simulink model "sl_groundvehicleDynamics"  (R2022b)
settings: Solver=ode45  StartTime=0.0  StopTime=50  RelTol=1e-5  EnableMultiTasking=on
libraries: simulink x4, mobileRoboticsLib x3, simulink_extras x2
settings Model: Creator=sriramn  LastModifiedBy=n10474056
settings SolverCC: ZeroCrossAlgorithm=Adaptive  AlgebraicLoopSolver=TrustRegion
settings DataIOCC: LimitDataPoints=on  SaveFormat=Array  ReturnWorkspaceOutputs=off
settings OptimizationCC: LifeSpan=inf
settings DebuggingCC: SolverPrmCheckMsg=warning  UnconnectedInputMsg=warning  UnconnectedOutputMsg=warning  UnconnectedLineMsg=warning  AllowSymbolicDim=off  SFUnexpectedBacktrackingDiag=warning  SFNoUnconditionalDefaultTransitionDiag=warning  SFExecutionAtInitializationDiag=none  SFMachineParentedDataDiag=warning  ArithmeticOperatorsInVariantConditions=warning
settings HardwareCC: ProdBitPerPointer=32  ProdBitPerSizeT=32  ProdBitPerPtrDiffT=32  ProdLargestAtomicFloat=None  ProdIntDivRoundTo=Undefined  ProdEndianess=Unspecified  ProdWordSize=32  ProdHWDeviceType=32-bit Generic
settings ModelReferenceCC: EnableRefExpFcnMdlSchedulingChecks=on  ModelReferenceMinAlgLoopOccurrences=on  PropagateSignalLabelsOutOfModel=off
settings SFSimCC: SimUseLocalCustomCode=off  CustomCodeUndefinedFunction=UseInterfaceOnly
settings RTWCC: RTWUseLocalCustomCode=off
settings CodeAppCC: StateflowObjectComments=on
settings GRTTargetCC: TargetLangStandard=C89/C90 (ANSI)
settings ConfigComp: CovMetricSettings=dw  CovSaveCumulativeToWorkspaceVar=on  CovSaveSingleToWorkspaceVar=on  CovExternalEMLEnable=off  CovSFcnEnable=off
settings SimscapeCC: SimscapeNormalizeSystem=off
settings ConfigurationSet: Description=SimMechanics 2G
settings ExplorerConfigSet: InternalSimMechanicsExplorerSettings="<ExplorerConfiguration><canonicalview>planar_xy</canonicalview><AnimationSetting><BasePlaybackSpeed>1.0</BasePlaybackSpeed><PlaybackSpeedFactor>1.0</PlaybackSpeedFactor></AnimationSetting><TilePanel><TileInfo><Tiles Columns=\"1\" Count=\"1\" Rows=\"1\"><Column Left=\"2\" Weight=\"1\"/><Column Left=\"1628\"/><Row Top=\"2\" Weight=\"1\"/><Row Top=\"1072\"/><Tile Height=\"1\" Width=\"1\" X=\"0\" Y=\"0\"/></Tiles></TileInfo><SceneInfo><SceneViewer><BGColor><R>0.60000002384185791</R><G>0.60000002384185791</G><B>0.60000002384185791</B></BGColor><Camera><Position><X>0.22951840878551699</X><Y>0.32651610611526627</Y><Z>-0.27215421354393321</Z></Position><Center><X>-0.15775714411666431</X><Y>-0.15462825985839526</Y><Z>0.065702552916005602</Z></Center><Up><X>-0.56030137557930915</X><Y>0.72817587161684794</Y><Z>0.39474329445726858</Z></Up><Left>-0.21481383955700509</Left><Right>0.21481383955700509</Right><Bottom>-0.27569784609469139</Bottom><Top>0.27569784609469139</Top></Camera></SceneViewer></SceneInfo></TilePanel></ExplorerConfiguration>"

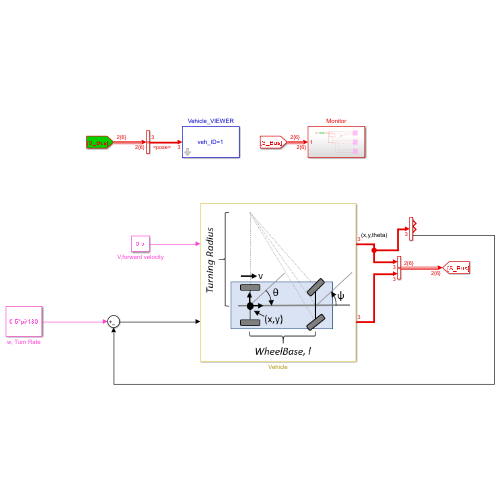
[thumbnail: Simulink's stored preview of the top-level diagram]
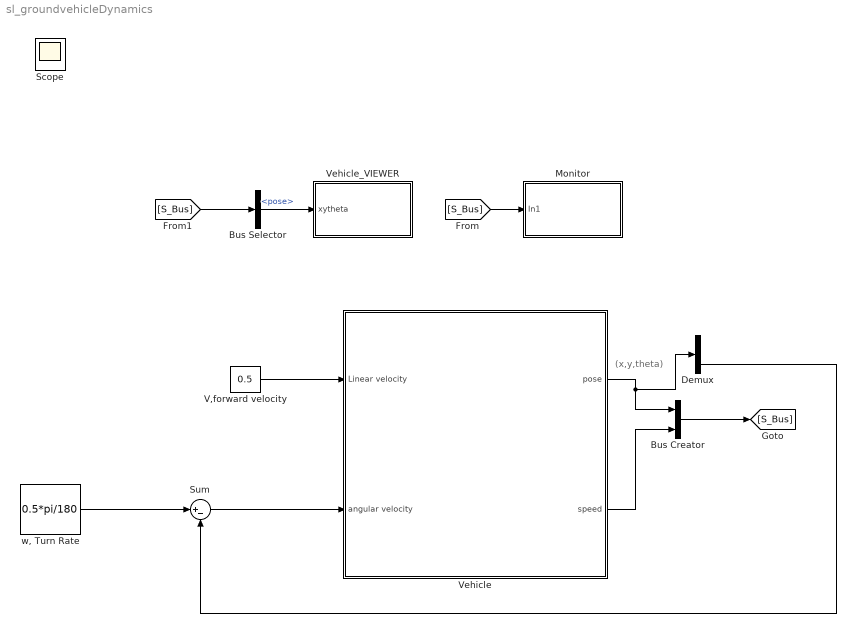
== system sl_groundvehicleDynamics ==
  note: (x,y,theta)
  Bus Creator : BusCreator  Inputs=2
  Bus Selector : BusSelector  OutputSignals=pose
  Demux : Demux  Outputs=3
  Monitor : Subsystem
  Sum : Sum  Inputs=|+-
  V,forward velocity : Constant  Value=0.5
  Vehicle : Subsystem
      mask Display: image('$imagefile'); % Use "Edit Image" on toolstrip to change.
  Vehicle_VIEWER : Subsystem  mask{wp_mat=[-100, 100;-100, 100]', veh_ID_num=1, veh_init_xytheta=[0 0 0], Ts=0.5}
      mask prompts: wp_mat "Waypoint matrix for arena [x_col, y_col] (m)"; veh_ID_num "Vehicle ID number"; veh_init_xytheta "Initial pose [x,y,theta]"; Ts "Sample time for updating animation (secs)"
      mask TypeOptions veh_ID_num: 1 | 2 | 3 | 4
      mask DialogControl Control2 Prompt: Animate simulation of Differential Drive Robot (DDR)
      mask Display: fprintf('veh_ID=%d',veh_ID_num);
  "w, Turn Rate" : Constant  Value=0.5*pi/180
  Scope : Scope
  wires:
  [S_Bus] -> Monitor/1(In1)
  [S_Bus] -> Bus Selector/1
  V,forward velocity/1 -> Vehicle/1(Linear velocity)
  Vehicle/1(pose) -> Demux/1, Bus Creator/1
  Vehicle/2(speed) -> Bus Creator/2
  Bus Creator/1 -> [S_Bus]
  Bus Selector/1 -> Vehicle_VIEWER/1(xytheta)  "<pose>"
  "w, Turn Rate"/1 -> Sum/1
  Sum/1 -> Vehicle/2(angular velocity)
  Demux/3 -> Sum/2

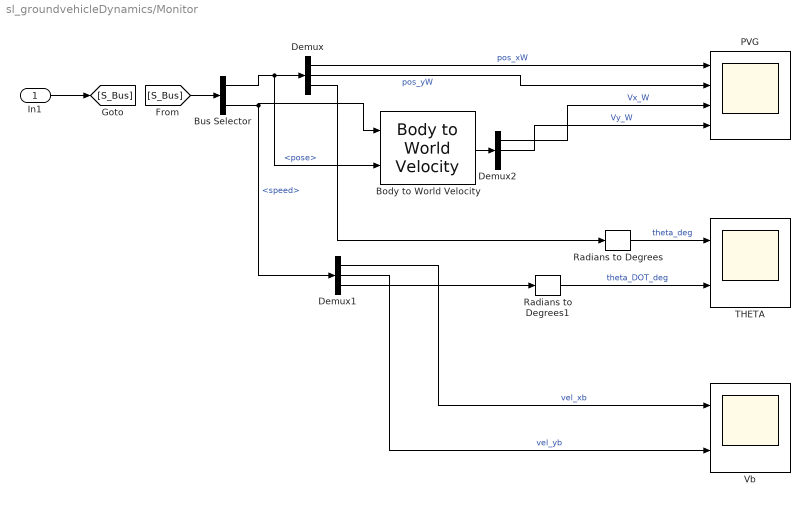
== system sl_groundvehicleDynamics/Monitor ==
  In1 : Inport
  Body to World Velocity : mobileRoboticsLib/Utilities/Body to World Velocity
      settings: SourceProductName=Mobile Robotics Simulation Toolbox
  Bus Selector : BusSelector  OutputSignals=pose,speed
  Demux : Demux  Outputs=3
  Demux1 : Demux  Outputs=3
  Demux2 : Demux  Outputs=3
  PVG : Scope  NumInputPorts=4
  Radians to Degrees : simulink_extras/Transformations/Radians to Degrees
  Radians to Degrees1 : simulink_extras/Transformations/Radians to Degrees
  THETA : Scope  NumInputPorts=2
  Vb : Scope  NumInputPorts=2
  wires:
  In1/1 -> [S_Bus]
  [S_Bus] -> Bus Selector/1
  Demux/1 -> PVG/1  "pos_xW"
  Demux/2 -> PVG/2  "pos_yW"
  Radians to Degrees1/1 -> THETA/2  "theta_DOT_deg"
  Radians to Degrees/1 -> THETA/1  "theta_deg"
  Demux1/3 -> Radians to Degrees1/1
  Demux/3 -> Radians to Degrees/1
  Bus Selector/1 -> Body to World Velocity/2, Demux/1  "<pose>"
  Bus Selector/2 -> Demux1/1, Body to World Velocity/1  "<speed>"
  Body to World Velocity/1 -> Demux2/1
  Demux2/1 -> PVG/3  "Vx_W"
  Demux2/2 -> PVG/4  "Vy_W"
  Demux1/1 -> Vb/1  "vel_xb"
  Demux1/2 -> Vb/2  "vel_yb"

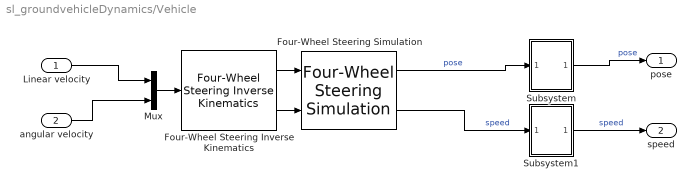
== system sl_groundvehicleDynamics/Vehicle ==
  Linear velocity : Inport
  angular velocity : Inport  Port=2
  Four-Wheel Steering Inverse Kinematics : mobileRoboticsLib/Kinematic Models/Four-Wheel Steering/Four-Wheel Steering Inverse Kinematics  wheelRadius=0.1  frontWheelDist=0.25  rearWheelDist=0.25  ikMode=Front Steering
      settings: SourceProductName=Mobile Robotics Simulation Toolbox
  Four-Wheel Steering Simulation : mobileRoboticsLib/Kinematic Models/Four-Wheel Steering/Four-Wheel Steering Simulation  wheelRadius=0.1  frontWheelDist=0.25  rearWheelDist=0.25  initX=0  initY=0  initAngle=0  Ts=0.05
      settings: SourceProductName=Mobile Robotics Simulation Toolbox
  Mux : Mux  Inputs=2
  Subsystem : Subsystem
  Subsystem1 : Subsystem
  pose : Outport  VectorParamsAs1DForOutWhenUnconnected=off
  speed : Outport  Port=2
  wires:
  angular velocity/1 -> Mux/2
  Linear velocity/1 -> Mux/1
  Mux/1 -> Four-Wheel Steering Inverse Kinematics/1
  Four-Wheel Steering Simulation/1 -> Subsystem/1(In1)  "pose"
  Four-Wheel Steering Simulation/2 -> Subsystem1/1(In1)  "speed"
  Four-Wheel Steering Inverse Kinematics/1 -> Four-Wheel Steering Simulation/1
  Four-Wheel Steering Inverse Kinematics/2 -> Four-Wheel Steering Simulation/2
  Subsystem/1(pose) -> pose/1  "pose"
  Subsystem1/1(speed) -> speed/1  "speed"

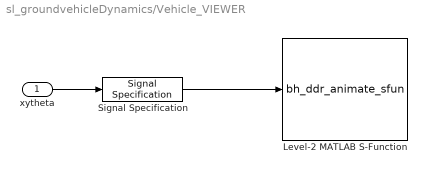
== system sl_groundvehicleDynamics/Vehicle_VIEWER ==
  xytheta : Inport
  Level-2 MATLAB S-Function : M-S-Function  FunctionName=bh_ddr_animate_sfun  Parameters=Ts, wp_mat, veh_ID_num, veh_init_xytheta
  Signal Specification : SignalSpecification  Dimensions=3
  wires:
  xytheta/1 -> Signal Specification/1
  Signal Specification/1 -> Level-2 MATLAB S-Function/1

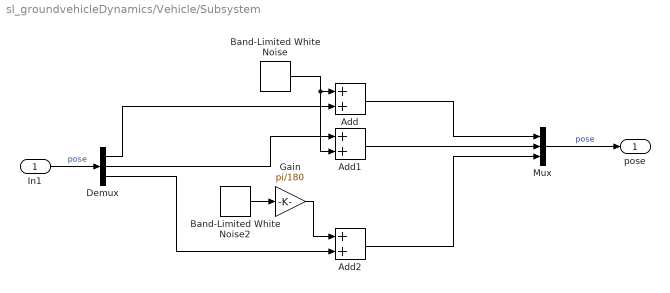
== system sl_groundvehicleDynamics/Vehicle/Subsystem ==
  In1 : Inport
  Add : Sum
  Add1 : Sum
  Add2 : Sum
  Band-Limited White Noise : simulink/Sources/Band-Limited White Noise  Cov=[0.001]  Ts=0.1  seed=[23341]
  Band-Limited White Noise2 : simulink/Sources/Band-Limited White Noise  Cov=[0.41]  Ts=0.1  seed=[23341]
  Demux : Demux  Outputs=3
  Gain : Gain  Gain=pi/180
  Mux : Mux  Inputs=3
  pose : Outport
  wires:
  Add1/1 -> Mux/2
  Add2/1 -> Mux/3
  Demux/2 -> Add1/1
  Band-Limited White Noise2/1 -> Gain/1
  Demux/3 -> Add2/2
  Band-Limited White Noise/1 -> Add1/2, Add/1
  In1/1 -> Demux/1  "pose"
  Demux/1 -> Add/2
  Gain/1 -> Add2/1
  Mux/1 -> pose/1  "pose"
  Add/1 -> Mux/1

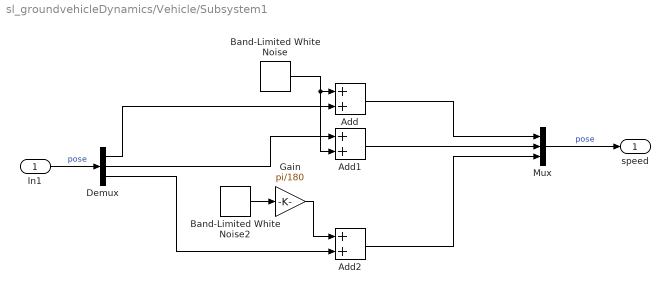
== system sl_groundvehicleDynamics/Vehicle/Subsystem1 ==
  In1 : Inport
  Add : Sum
  Add1 : Sum
  Add2 : Sum
  Band-Limited White Noise : simulink/Sources/Band-Limited White Noise  Cov=[0.001]  Ts=0.1  seed=[23341]
  Band-Limited White Noise2 : simulink/Sources/Band-Limited White Noise  Cov=[0.41]  Ts=0.1  seed=[23341]
  Demux : Demux  Outputs=3
  Gain : Gain  Gain=pi/180
  Mux : Mux  Inputs=3
  speed : Outport
  wires:
  Add1/1 -> Mux/2
  Add2/1 -> Mux/3
  Demux/2 -> Add1/1
  Band-Limited White Noise2/1 -> Gain/1
  Demux/3 -> Add2/2
  Band-Limited White Noise/1 -> Add1/2, Add/1
  In1/1 -> Demux/1  "pose"
  Demux/1 -> Add/2
  Gain/1 -> Add2/1
  Mux/1 -> speed/1  "pose"
  Add/1 -> Mux/1
